simulink model "SinusWaveModelling"  (R2024b)
settings: Solver=VariableStepAuto  StartTime=0.0  StopTime=2  RelTol=1e-3
undefined symbols (not defined in the file or in its folder): j
settings Model: Creator=castl  LastModifiedBy=castl

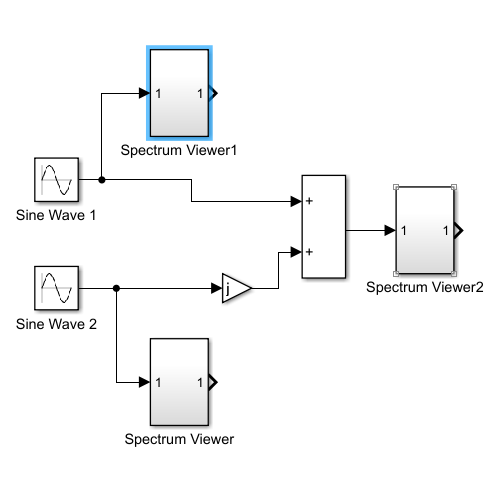
[thumbnail: Simulink's stored preview of the top-level diagram]
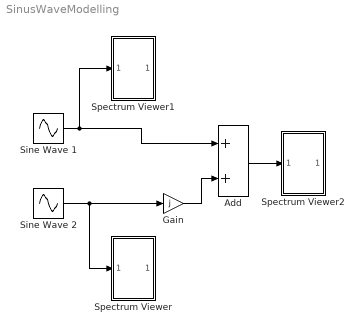
== system SinusWaveModelling ==
  Add : Sum
  Gain : Gain  Gain=j
  Sine Wave 1 : Sin  Frequency=2*pi*(22000)  Phase=pi/2  SampleTime=0
  Sine Wave 2 : Sin  Frequency=2*pi*3000  Phase=4  SampleTime=0
  Spectrum Viewer : Subsystem
  Spectrum Viewer1 : Subsystem
  Spectrum Viewer2 : Subsystem
  wires:
  Add/1 -> Spectrum Viewer2/1(In1)
  Sine Wave 1/1 -> Add/1, Spectrum Viewer1/1(In1)
  Gain/1 -> Add/2
  Sine Wave 2/1 -> Spectrum Viewer/1(In1), Gain/1

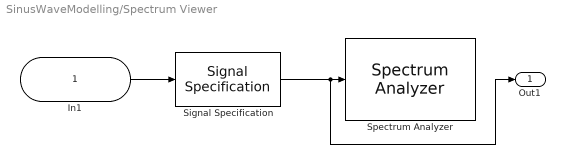
== system SinusWaveModelling/Spectrum Viewer ==
  In1 : Inport
  Signal Specification : SignalSpecification  SampleTime=1/16e4
  Spectrum Analyzer : SpectrumAnalyzer  WindowPosition=[1659.000000,375.000000,800.000000,782.000000,]  ScopeFrameLocation=window  Method=Welch  AxesScaling=Manual  FrequencyResolutionMethod=Window length  FrequencySpan=Span and center frequency  Span=160000  StartFrequency=-80000  StopFrequency=80000  OverlapPercent=6.25  AveragingMethod=Running  SpectralAverages=200  SpectrumUnits=Watts  YLimits=[-0.019423423539448113,0.07466740249489141]  SelectedToolstripTab=spectrumAnalyzerToolstrip.spectrumTab  AllowFFTLengthLessThanSamplesPerUpdate=on  DefaultConfigurationName=spbscopes.SpectrumAnalyzerBlockCfg  IsFrequencyInputMode=0  FrequencyVectorPort=0  FrequencyVectorFromPort=0  FrequencyInputRBWPort=0  FrequencyInputRBWFromPort=0
  Out1 : Outport
  wires:
  In1/1 -> Signal Specification/1
  Signal Specification/1 -> Out1/1, Spectrum Analyzer/1

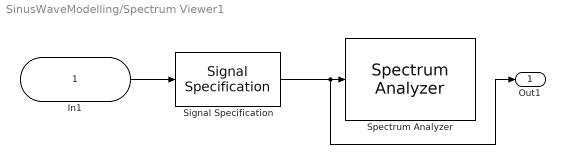
== system SinusWaveModelling/Spectrum Viewer1 ==
  In1 : Inport
  Signal Specification : SignalSpecification  SampleTime=1/16e4
  Spectrum Analyzer : SpectrumAnalyzer  WindowPosition=[860.000000,441.000000,800.000000,782.000000,]  ScopeFrameLocation=window  Method=Welch  AxesScaling=Manual  FrequencyResolutionMethod=Window length  FrequencySpan=Span and center frequency  Span=160000  StartFrequency=-80000  StopFrequency=80000  OverlapPercent=6.25  AveragingMethod=Running  SpectralAverages=200  SpectrumUnits=Watts  YLimits=[-0.11013968516007862,0.44594244974112696]  SelectedToolstripTab=spectrumAnalyzerToolstrip.spectrumTab  AllowFFTLengthLessThanSamplesPerUpdate=on  DefaultConfigurationName=spbscopes.SpectrumAnalyzerBlockCfg  IsFrequencyInputMode=0  FrequencyVectorPort=0  FrequencyVectorFromPort=0  FrequencyInputRBWPort=0  FrequencyInputRBWFromPort=0
  Out1 : Outport
  wires:
  In1/1 -> Signal Specification/1
  Signal Specification/1 -> Out1/1, Spectrum Analyzer/1

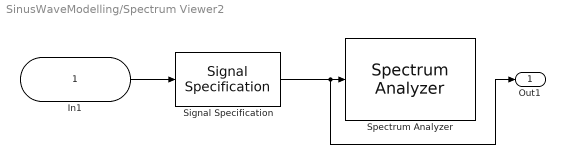
== system SinusWaveModelling/Spectrum Viewer2 ==
  In1 : Inport
  Signal Specification : SignalSpecification  SampleTime=1/16e4
  Spectrum Analyzer : SpectrumAnalyzer  WindowPosition=[465.000000,423.000000,800.000000,782.000000,]  ScopeFrameLocation=window  Method=Welch  AxesScaling=Manual  FrequencyResolutionMethod=Window length  FrequencySpan=Span and center frequency  Span=160000  StartFrequency=-80000  StopFrequency=80000  OverlapPercent=6.25  AveragingMethod=Running  SpectralAverages=200  SpectrumUnits=Watts  YLimits=[-0.10809447526868737,1.203408955641157]  SelectedToolstripTab=spectrumAnalyzerToolstrip.spectrumTab  AllowFFTLengthLessThanSamplesPerUpdate=on  DefaultConfigurationName=spbscopes.SpectrumAnalyzerBlockCfg  IsFrequencyInputMode=0  FrequencyVectorPort=0  FrequencyVectorFromPort=0  FrequencyInputRBWPort=0  FrequencyInputRBWFromPort=0
  Out1 : Outport
  wires:
  In1/1 -> Signal Specification/1
  Signal Specification/1 -> Out1/1, Spectrum Analyzer/1
